simulink model "Suspension"  (R2020a)
settings: Solver=VariableStepAuto  StartTime=0.0  StopTime=50  RelTol=1e-3
values from neighbouring files (symbols this model uses):
  b1 = 350    [matlab.mat]
  b2 = 15020    [matlab.mat]
  k1 = 80000    [matlab.mat]
  k2 = 500000    [matlab.mat]
  m1 = 2500    [matlab.mat]
  m2 = 320    [matlab.mat]
settings Model: Creator=intel  LastModifiedBy=intel

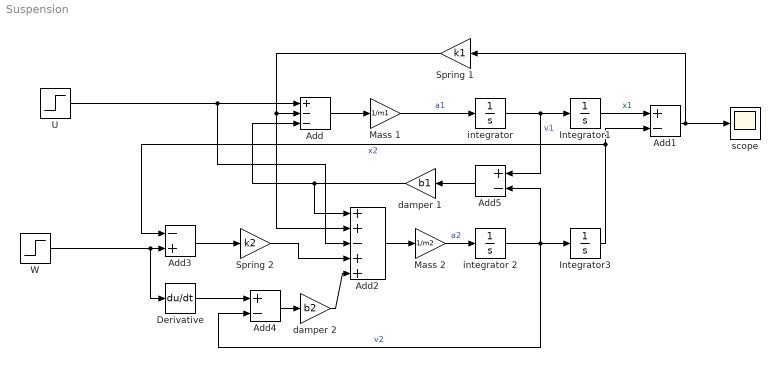
== system Suspension ==
  Add : Sum  Inputs=+--
  Add1 : Sum  Inputs=+-
  Add2 : Sum  Inputs=++-++
  Add3 : Sum  Inputs=-+
  Add4 : Sum  Inputs=+-
  Add5 : Sum  Inputs=+-
  Derivative : Derivative
  Integrator1 : Integrator
  Integrator3 : Integrator
  Mass 1 : Gain  Gain=1/m1
  Mass 2 : Gain  Gain=1/m2
  Spring 1 : Gain  Gain=k1
  Spring 2 : Gain  Gain=k2
  U : Step  Time=0  SampleTime=0
  W : Step  Time=0  After=0  SampleTime=0
  damper 1 : Gain  Gain=b1
  damper 2 : Gain  Gain=b2
  "integrator " : Integrator
  integrator 2 : Integrator
  scope : Scope
  wires:
  U/1 -> Add2/3, Add/1
  Add/1 -> Mass 1/1
  Mass 1/1 -> "integrator "/1  "a1"
  "integrator "/1 -> Add5/1, Integrator1/1  "v1"
  Integrator1/1 -> Add1/1  "x1"
  Add1/1 -> Spring 1/1, scope/1
  Add2/1 -> Mass 2/1
  Add3/1 -> Spring 2/1
  Spring 1/1 -> Add2/2, Add/2
  Mass 2/1 -> integrator 2/1  "a2"
  Integrator3/1 -> Add3/1, Add1/2  "x2"
  Spring 2/1 -> Add2/4
  Add4/1 -> damper 2/1
  W/1 -> Derivative/1, Add3/2
  damper 2/1 -> Add2/5
  integrator 2/1 -> Add4/2, Add5/2, Integrator3/1  "v2"
  Add5/1 -> damper 1/1
  damper 1/1 -> Add2/1, Add/3
  Derivative/1 -> Add4/1
